simulink model "Four_DG_MG_PrimaryOnly"  (R2021b)
settings: Solver=ode23tb  StartTime=0.0  StopTime=5  RelTol=1e-3
model workspace (MAT data in the model file):
  Ts : Simulink.Parameter (value not decoded)
  secondary_on : Simulink.Parameter (value not decoded)
values from neighbouring files (symbols this model uses):
  a12 = 0    [Four_DG_MG_PrimaryOnlyScript.m]    (also in MPC_MG_script_raw_dmpc.m; MPC_MG_secondary_script.m)
  a14 = 0    [Four_DG_MG_PrimaryOnlyScript.m]    (also in MPC_MG_script_raw_dmpc.m; MPC_MG_secondary_script.m)
  a21 = 1    [Four_DG_MG_PrimaryOnlyScript.m]    (also in MPC_MG_script_raw_dmpc.m; MPC_MG_secondary_script.m)
  a23 = 0    [Four_DG_MG_PrimaryOnlyScript.m]    (also in MPC_MG_script_raw_dmpc.m; MPC_MG_secondary_script.m)
  a32 = 1    [Four_DG_MG_PrimaryOnlyScript.m]    (also in MPC_MG_script_raw_dmpc.m; MPC_MG_secondary_script.m)
  a34 = 0    [Four_DG_MG_PrimaryOnlyScript.m]    (also in MPC_MG_script_raw_dmpc.m; MPC_MG_secondary_script.m)
  a41 = 1    [Four_DG_MG_PrimaryOnlyScript.m]    (also in MPC_MG_script_raw_dmpc.m; MPC_MG_secondary_script.m)
  a43 = 0    [Four_DG_MG_PrimaryOnlyScript.m]    (also in MPC_MG_script_raw_dmpc.m; MPC_MG_secondary_script.m)
  b1v = 1    [Four_DG_MG_PrimaryOnlyScript.m]    (also in MPC_MG_script_raw_dmpc.m; MPC_MG_secondary_script.m; MPG_MG_July.m; MPG_MG_freq_script.m)
  b1w = 1    [Four_DG_MG_PrimaryOnlyScript.m]    (also in MPC_MG_script_raw_dmpc.m; MPC_MG_secondary_script.m; MPG_MG_July.m; MPG_MG_freq_script.m)
  b2v = 0    [Four_DG_MG_PrimaryOnlyScript.m]    (also in MPC_MG_script_raw_dmpc.m; MPC_MG_secondary_script.m; MPG_MG_July.m; MPG_MG_freq_script.m)
  b2w = 0    [Four_DG_MG_PrimaryOnlyScript.m]    (also in MPC_MG_script_raw_dmpc.m; MPC_MG_secondary_script.m; MPG_MG_July.m; MPG_MG_freq_script.m)
  b3v = 0    [Four_DG_MG_PrimaryOnlyScript.m]    (also in MPC_MG_script_raw_dmpc.m; MPC_MG_secondary_script.m; MPG_MG_July.m; MPG_MG_freq_script.m)
  b3w = 0    [Four_DG_MG_PrimaryOnlyScript.m]    (also in MPC_MG_script_raw_dmpc.m; MPC_MG_secondary_script.m; MPG_MG_July.m; MPG_MG_freq_script.m)
  b4v = 0    [Four_DG_MG_PrimaryOnlyScript.m]    (also in MPC_MG_script_raw_dmpc.m; MPC_MG_secondary_script.m; MPG_MG_July.m; MPG_MG_freq_script.m)
  b4w = 0    [Four_DG_MG_PrimaryOnlyScript.m]    (also in MPC_MG_script_raw_dmpc.m; MPC_MG_secondary_script.m; MPG_MG_July.m; MPG_MG_freq_script.m)
  C_f = 50e-6    (= 5e-05)    [Four_DG_MG_PrimaryOnlyScript.m]    (also in MPC_MG_script.m; MPC_MG_script_raw_dmpc.m; MPC_MG_secondary_script.m; MPG_MG_July.m)
  cf = 60    [Four_DG_MG_PrimaryOnlyScript.m]    (also in MPC_MG_script_raw_dmpc.m = 40; MPC_MG_secondary_script.m = 40; MPG_MG_July.m = 100; MPG_MG_freq_script.m = 100)
  cv = 60    [Four_DG_MG_PrimaryOnlyScript.m]    (also in MPC_MG_script_raw_dmpc.m = 40; MPC_MG_secondary_script.m = 40; MPG_MG_July.m = 100; MPG_MG_freq_script.m = 100)
  F = 1    [Four_DG_MG_PrimaryOnlyScript.m]    (also in dmpc.m = zeros(9,1))
  K_i1 = 420    [Four_DG_MG_PrimaryOnlyScript.m]
  K_i2 = K_i1    (= 420)    [Four_DG_MG_PrimaryOnlyScript.m]
  K_i3 = 390    [Four_DG_MG_PrimaryOnlyScript.m]
  K_i4 = K_i3    (= 390)    [Four_DG_MG_PrimaryOnlyScript.m]
  K_ii1 = 5e3    (= 5000)    [Four_DG_MG_PrimaryOnlyScript.m]
  K_ii2 = K_ii1    (= 5000)    [Four_DG_MG_PrimaryOnlyScript.m]
  K_ii3 = 16e3    (= 16000)    [Four_DG_MG_PrimaryOnlyScript.m]
  K_ii4 = K_ii3    (= 16000)    [Four_DG_MG_PrimaryOnlyScript.m]
  K_p1 = 0.1    [Four_DG_MG_PrimaryOnlyScript.m]
  K_p2 = K_p1    (= 0.1)    [Four_DG_MG_PrimaryOnlyScript.m]
  K_p3 = 0.05    [Four_DG_MG_PrimaryOnlyScript.m]
  K_p4 = K_p3    (= 0.05)    [Four_DG_MG_PrimaryOnlyScript.m]
  K_pi1 = 5    [Four_DG_MG_PrimaryOnlyScript.m]
  K_pi2 = K_pi1    (= 5)    [Four_DG_MG_PrimaryOnlyScript.m]
  K_pi3 = 10.5    [Four_DG_MG_PrimaryOnlyScript.m]
  K_pi4 = K_pi3    (= 10.5)    [Four_DG_MG_PrimaryOnlyScript.m]
  L_f = 1.35e-3    (= 0.00135)    [Four_DG_MG_PrimaryOnlyScript.m]    (also in MPC_MG_script.m; MPC_MG_script_raw_dmpc.m; MPC_MG_secondary_script.m; MPG_MG_July.m)
  L_in1 = 0.35e-3    (= 0.00035)    [Four_DG_MG_PrimaryOnlyScript.m]    (also in MPC_MG_script.m; MPC_MG_script_raw_dmpc.m; MPC_MG_secondary_script.m; MPG_MG_July.m)
  L_in2 = 0.35e-3    (= 0.00035)    [Four_DG_MG_PrimaryOnlyScript.m]    (also in MPC_MG_script.m; MPC_MG_script_raw_dmpc.m; MPC_MG_secondary_script.m; MPG_MG_July.m)
  L_in3 = 0.35e-3    (= 0.00035)    [Four_DG_MG_PrimaryOnlyScript.m]    (also in MPC_MG_script.m; MPC_MG_script_raw_dmpc.m; MPC_MG_secondary_script.m; MPG_MG_July.m)
  L_in4 = 0.35e-3    (= 0.00035)    [Four_DG_MG_PrimaryOnlyScript.m]    (also in MPC_MG_script.m; MPC_MG_script_raw_dmpc.m; MPC_MG_secondary_script.m; MPG_MG_July.m)
  lo_co = 0.2    [Four_DG_MG_PrimaryOnlyScript.m]    (also in MPC_MG_script.m = 0.05; MPC_MG_script_raw_dmpc.m; MPC_MG_secondary_script.m = 0.08; MPG_MG_July.m = 0.15)
  m_p1 = 9.4e-5/droopDivide    (= 9.4e-05)    [Four_DG_MG_PrimaryOnlyScript.m]    (also in MPC_MG_script.m; MPC_MG_script_raw_dmpc.m; MPC_MG_secondary_script.m; MPG_MG_July.m)
  m_p2 = 9.4e-5/droopDivide    (= 9.4e-05)    [Four_DG_MG_PrimaryOnlyScript.m]    (also in MPC_MG_script.m; MPC_MG_script_raw_dmpc.m; MPC_MG_secondary_script.m; MPG_MG_July.m)
  m_p3 = 12.5e-5/droopDivide    (= 0.000125)    [Four_DG_MG_PrimaryOnlyScript.m]    (also in MPC_MG_script.m; MPC_MG_script_raw_dmpc.m; MPC_MG_secondary_script.m; MPG_MG_July.m)
  m_p4 = 12.5e-5/droopDivide    (= 0.000125)    [Four_DG_MG_PrimaryOnlyScript.m]    (also in MPC_MG_script.m; MPC_MG_script_raw_dmpc.m; MPC_MG_secondary_script.m; MPG_MG_July.m)
  n_q1 = 1.3e-3/droopDivide2    (= 0.00013)    [Four_DG_MG_PrimaryOnlyScript.m]    (also in MPC_MG_script.m; MPC_MG_script_raw_dmpc.m; MPC_MG_secondary_script.m; MPG_MG_July.m)
  n_q2 = 1.3e-3/droopDivide2    (= 0.00013)    [Four_DG_MG_PrimaryOnlyScript.m]    (also in MPC_MG_script.m; MPC_MG_script_raw_dmpc.m; MPC_MG_secondary_script.m; MPG_MG_July.m)
  n_q3 = 1.5e-3/droopDivide2    (= 0.00015)    [Four_DG_MG_PrimaryOnlyScript.m]    (also in MPC_MG_script.m; MPC_MG_script_raw_dmpc.m; MPC_MG_secondary_script.m; MPG_MG_July.m)
  n_q4 = 1.5e-3/droopDivide2    (= 0.00015)    [Four_DG_MG_PrimaryOnlyScript.m]    (also in MPC_MG_script.m; MPC_MG_script_raw_dmpc.m; MPC_MG_secondary_script.m; MPG_MG_July.m)
  pq_gain = 3/2    (= 1.5)    [Four_DG_MG_PrimaryOnlyScript.m]
  R_f = 0.1    [Four_DG_MG_PrimaryOnlyScript.m]    (also in MPC_MG_script.m; MPC_MG_script_raw_dmpc.m; MPC_MG_secondary_script.m; MPG_MG_July.m)
  R_in1 = 0.03    [Four_DG_MG_PrimaryOnlyScript.m]    (also in MPC_MG_script.m; MPC_MG_script_raw_dmpc.m; MPC_MG_secondary_script.m; MPG_MG_July.m)
  R_in2 = 0.03    [Four_DG_MG_PrimaryOnlyScript.m]    (also in MPC_MG_script.m; MPC_MG_script_raw_dmpc.m; MPC_MG_secondary_script.m; MPG_MG_July.m)
  R_in3 = 0.03    [Four_DG_MG_PrimaryOnlyScript.m]    (also in MPC_MG_script.m; MPC_MG_script_raw_dmpc.m; MPC_MG_secondary_script.m; MPG_MG_July.m)
  R_in4 = 0.03    [Four_DG_MG_PrimaryOnlyScript.m]    (also in MPC_MG_script.m; MPC_MG_script_raw_dmpc.m; MPC_MG_secondary_script.m; MPG_MG_July.m)
  secondary = 1    [Four_DG_MG_PrimaryOnlyScript.m]
  secondary2 = 1    [Four_DG_MG_PrimaryOnlyScript.m]
  time_thresh = 0.6    [Four_DG_MG_PrimaryOnlyScript.m]    (also in MPC_MG_script_raw_dmpc.m = 1.5; MPC_MG_secondary_script.m = 2; MPG_MG_July.m = 0.5; MPG_MG_freq_script.m = 0.5)
  Ts = 10e-6    (= 1e-05)    [Four_DG_MG_PrimaryOnlyScript.m]    (also in MPC_MG_script.m; MPC_MG_script_raw_dmpc.m; MPC_MG_secondary_script.m; MPG_MG_July.m)
  V_nom = 220*sqrt(2)    [Four_DG_MG_PrimaryOnlyScript.m]    (also in MPC_MG_script.m; MPC_MG_script_raw_dmpc.m; MPC_MG_secondary_script.m; MPG_MG_July.m)
  Vdc = 600    [Four_DG_MG_PrimaryOnlyScript.m]    (also in MPC_MG_script.m; MPC_MG_script_raw_dmpc.m; MPC_MG_secondary_script.m; MPG_MG_July.m)
  w_nom = 2*pi*50    (= 314.159265359)    [Four_DG_MG_PrimaryOnlyScript.m]    (also in MPC_MG_script.m; MPC_MG_script_raw_dmpc.m; MPC_MG_secondary_script.m; MPG_MG_July.m)
undefined symbols (not defined in the file or in its folder): K_d
libraries: slpidlib x16, spsThreePhaseSeriesRLCBranchLib x15, spsabctodq0Lib x13, spsThreePhaseVIMeasurementLib x12, eeGeneralControl x8, spsOnDelayLib x8, spsPMUPLLBasedPositiveSequenceLib x4, eePwmGeneratorTwoLevel x4, spsdq0toabcLib x4, spsDCVoltageSourceLib x4, spsSeriesRLCBranchLib x4, spsTwoLevelConverterLib x4
(part 4 of 4)

== system Four_DG_MG_PrimaryOnly/Voltage Source Inverter 3/Controller/PQ calculator ==
  Vod : Inport
  Voq : Inport  Port=2
  Iod : Inport  Port=3
  Ioq : Inport  Port=4
  Product{,1..3} (4 alike) : Product
  Sum10 : Sum  Inputs=|++
  Sum11 : Sum  Inputs=|+-
  p_hat : Outport
  q_hat : Outport  Port=2
  wires:
  Product3/1 -> Sum11/2
  Product1/1 -> Sum10/2
  Voq/1 -> Product3/1, Product1/1
  Iod/1 -> Product/2, Product3/2
  Product2/1 -> Sum11/1
  Ioq/1 -> Product1/2, Product2/2
  Product/1 -> Sum10/1
  Vod/1 -> Product/1, Product2/1
  Sum11/1 -> q_hat/1  "q_hat"
  Sum10/1 -> p_hat/1  "p_hat"

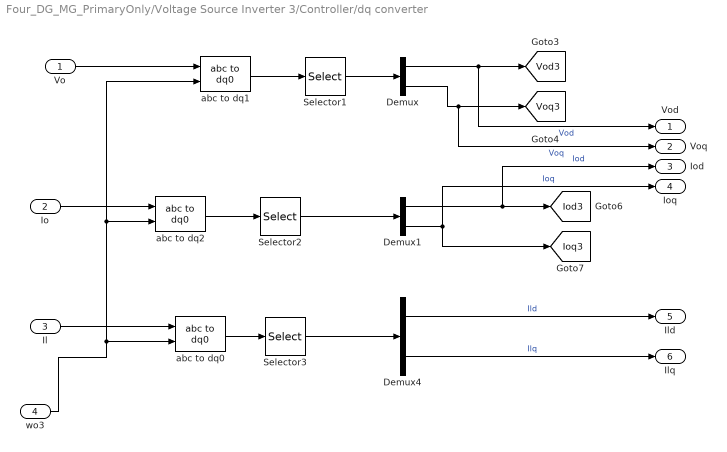
== system Four_DG_MG_PrimaryOnly/Voltage Source Inverter 3/Controller/dq converter ==
  Vo : Inport
  Io : Inport  Port=2
  Il : Inport  Port=3
  wo3 : Inport  Port=4
  Demux : Demux  Outputs=2
  Demux1 : Demux  Outputs=2
  Demux4 : Demux  Outputs=2
  Selector1 : Selector  InputPortWidth=3  IndexOptions=Index vector (dialog)  Indices=[1 2]  OutputSizes=1
  Selector2 : Selector  InputPortWidth=3  IndexOptions=Index vector (dialog)  Indices=[1 2]  OutputSizes=1
  Selector3 : Selector  InputPortWidth=3  IndexOptions=Index vector (dialog)  Indices=[1 2]  OutputSizes=1
  abc to dq0 : spsabctodq0Lib/abc to dq0  Alignment=90 degrees behind phase A axis
  abc to dq1 : spsabctodq0Lib/abc to dq0  Alignment=90 degrees behind phase A axis
  abc to dq2 : spsabctodq0Lib/abc to dq0  Alignment=90 degrees behind phase A axis
  Vod : Outport
  Voq : Outport  Port=2
  Iod : Outport  Port=3
  Ioq : Outport  Port=4
  Ild : Outport  Port=5
  Ilq : Outport  Port=6
  tag scope: Iod3=global, Ioq3=global, Vod3=global, Voq3=global
  wires:
  Vo/1 -> abc to dq1/1
  Demux/1 -> Vod/1, [Vod3]  "Vod"
  Demux1/1 -> Iod/1, [Iod3]  "Iod"
  Selector3/1 -> Demux4/1
  Demux/2 -> Voq/1, [Voq3]  "Voq"
  Selector1/1 -> Demux/1
  wo3/1 -> abc to dq0/2, abc to dq2/2, abc to dq1/2
  abc to dq2/1 -> Selector2/1
  abc to dq0/1 -> Selector3/1
  Demux1/2 -> Ioq/1, [Ioq3]  "Ioq"
  Demux4/1 -> Ild/1  "Ild"
  abc to dq1/1 -> Selector1/1
  Selector2/1 -> Demux1/1
  Io/1 -> abc to dq2/1
  Il/1 -> abc to dq0/1
  Demux4/2 -> Ilq/1  "Ilq"

== system Four_DG_MG_PrimaryOnly/Voltage Source Inverter 4/Controller/Droop for secondary control ==
  P : Inport
  Q : Inport  Port=2
  w_nom : Inport  Port=3
  V_nom : Inport  Port=4
  Gain4 : Gain  Gain=n_q4
  Gain5 : Gain  Gain=m_p4
  Integrator : Integrator  WrapState=on  WrappedStateUpperValue=2*pi  WrappedStateLowerValue=0
  Sum1 : Sum  Inputs=|+-
  Sum2 : Sum  Inputs=|+-
  Vod_s : Outport
  wo : Outport  Port=2
  tag scope: wot4=global
  wires:
  P/1 -> Gain5/1
  V_nom/1 -> Sum1/1
  Q/1 -> Gain4/1
  w_nom/1 -> Sum2/1
  Gain5/1 -> Sum2/2
  Gain4/1 -> Sum1/2
  Sum2/1 -> [wot4], Integrator/1  "w"
  Integrator/1 -> wo/1
  Sum1/1 -> Vod_s/1  "Vod_s"

== system Four_DG_MG_PrimaryOnly/Voltage Source Inverter 4/Controller/Low-pass filter ==
  p_hat : Inport
  q_hat : Inport  Port=2
  Low-Pass Filter (Discrete or Continuous) : eeGeneralControl/Low-Pass Filter (Discrete or Continuous)  K=1  T=lo_co  B=inf  A=-inf  init_option=Inherited from block input  x0=0  Ts=-1
  Low-Pass Filter (Discrete or Continuous)1 : eeGeneralControl/Low-Pass Filter (Discrete or Continuous)  K=1  T=lo_co  B=inf  A=-inf  init_option=Inherited from block input  x0=0  Ts=-1
  P : Outport
  Q : Outport  Port=2
  wires:
  q_hat/1 -> Low-Pass Filter (Discrete or Continuous)1/1
  Low-Pass Filter (Discrete or Continuous)1/1 -> Q/1  "Q"
  Low-Pass Filter (Discrete or Continuous)/1 -> P/1  "P"
  p_hat/1 -> Low-Pass Filter (Discrete or Continuous)/1

== system Four_DG_MG_PrimaryOnly/Voltage Source Inverter 4/Controller/PQ calculator ==
  Vod : Inport
  Voq : Inport  Port=2
  Iod : Inport  Port=3
  Ioq : Inport  Port=4
  Product{,1..3} (4 alike) : Product
  Sum10 : Sum  Inputs=|++
  Sum11 : Sum  Inputs=|+-
  p_hat : Outport
  q_hat : Outport  Port=2
  wires:
  Product3/1 -> Sum11/2
  Product1/1 -> Sum10/2
  Voq/1 -> Product3/1, Product1/1
  Iod/1 -> Product/2, Product3/2
  Product2/1 -> Sum11/1
  Ioq/1 -> Product1/2, Product2/2
  Product/1 -> Sum10/1
  Vod/1 -> Product/1, Product2/1
  Sum11/1 -> q_hat/1  "q_hat"
  Sum10/1 -> p_hat/1  "p_hat"

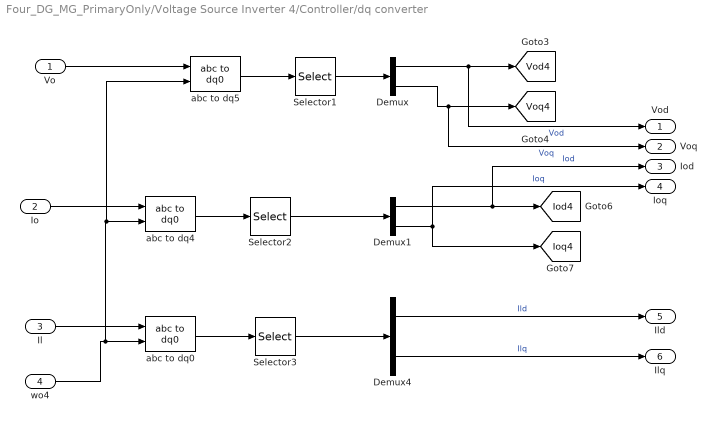
== system Four_DG_MG_PrimaryOnly/Voltage Source Inverter 4/Controller/dq converter ==
  Vo : Inport
  Io : Inport  Port=2
  Il : Inport  Port=3
  wo4 : Inport  Port=4
  Demux : Demux  Outputs=2
  Demux1 : Demux  Outputs=2
  Demux4 : Demux  Outputs=2
  Selector1 : Selector  InputPortWidth=3  IndexOptions=Index vector (dialog)  Indices=[1 2]  OutputSizes=1
  Selector2 : Selector  InputPortWidth=3  IndexOptions=Index vector (dialog)  Indices=[1 2]  OutputSizes=1
  Selector3 : Selector  InputPortWidth=3  IndexOptions=Index vector (dialog)  Indices=[1 2]  OutputSizes=1
  abc to dq0 : spsabctodq0Lib/abc to dq0  Alignment=90 degrees behind phase A axis
  abc to dq4 : spsabctodq0Lib/abc to dq0  Alignment=90 degrees behind phase A axis
  abc to dq5 : spsabctodq0Lib/abc to dq0  Alignment=90 degrees behind phase A axis
  Vod : Outport
  Voq : Outport  Port=2
  Iod : Outport  Port=3
  Ioq : Outport  Port=4
  Ild : Outport  Port=5
  Ilq : Outport  Port=6
  tag scope: Iod4=global, Ioq4=global, Vod4=global, Voq4=global
  wires:
  Vo/1 -> abc to dq5/1
  Demux/1 -> Vod/1, [Vod4]  "Vod"
  Demux1/1 -> Iod/1, [Iod4]  "Iod"
  wo4/1 -> abc to dq5/2, abc to dq4/2, abc to dq0/2
  Selector3/1 -> Demux4/1
  Demux/2 -> Voq/1, [Voq4]  "Voq"
  Selector1/1 -> Demux/1
  abc to dq4/1 -> Selector2/1
  abc to dq0/1 -> Selector3/1
  Demux1/2 -> Ioq/1, [Ioq4]  "Ioq"
  Demux4/1 -> Ild/1  "Ild"
  abc to dq5/1 -> Selector1/1
  Selector2/1 -> Demux1/1
  Io/1 -> abc to dq4/1
  Demux4/2 -> Ilq/1  "Ilq"
  Il/1 -> abc to dq0/1

== matlab function Four_DG_MG_PrimaryOnly/Voltage Source Inverter 1/Controller/MPC Secondary   ==
  data: invi input; wik_head output; invj1 input; invj2 input; wik output; delta_V output; delta_w output; deltaPhik output; Qik output; Pik output; Vik output; Vik_head output
function [wik_head,wik, delta_V, delta_w, deltaPhik, Qik, Pik, Vik, Vik_head] = fcn(invi, invj1, invj2)
Vl1 = invi(1);%trííc filter 
wl1 = invi(2);
Vo1 = invi(3); %phía output, cí star
wo1 = invi(4);
deltaPhi1 = invi(5);
P1 = invi(6);
Q1 = invi(7);
Tsec = 0.05;

%H = zeros(10,10);
%Initiate Hi, Fi, Ai, Aeqi, Bi, Beqi
%Initiate adjancancy matrix


syms w1k V1k deltaPhi1k P1k Q1k 
eqn1 = w1k == wl1 + m_p1*(P1k - P1); %neu prediction horizon > 1 thi doan nay se cong them deltaw cac kieu
eqn2 = V1k == Vl1 + n_q1*(Q1k - Q1);
eqn3 = deltaPhi1k == deltaPhi1 + Tsec*(w1k - wo1);
eqn4 = P1k == P1 + (V1k - Vl1)*Bi*Vo1*sin(deltaPhi1) + (deltaPhi1k - deltaPhi1)*Bi*Vl1*Vo1*cos(deltaPhi1);
eqn5 = Q1k == Q1 + (V1k - Vl1)*Bi*(2*Vl1 - Vo1*cos(deltaPhi1)) + (deltaPhi1k - deltaPhi1)*Bi*Vl1*Vo1*sin(deltaPhi1);

sol = solve([eqn1, eqn2, eqn3, eqn4, eqn5], [w1k, V1k, deltaPhi1k, P1k, Q1k]);
w1kSol = sol.w1k;
V1kSol = sol.V1k;
deltaPhi1kSol = sol.deltaPhi1k;
P1kSol = sol.P1k;
Q1kSol = sol.Q1k;



y = u;
